simulink model "ValvingPTO"  (R2024b)
settings: Solver=VariableStepAuto  StartTime=0.0  StopTime=10.0  RelTol=1e-3
values from neighbouring files (symbols this model uses):
  params = struct    [BranchAndBound.m]    (also in Optimization.m; Parameters.m = struct(); RectangularOptimization.m; RoundingPI.m)
settings Model: Creator=jackson  LastModifiedBy=jackson

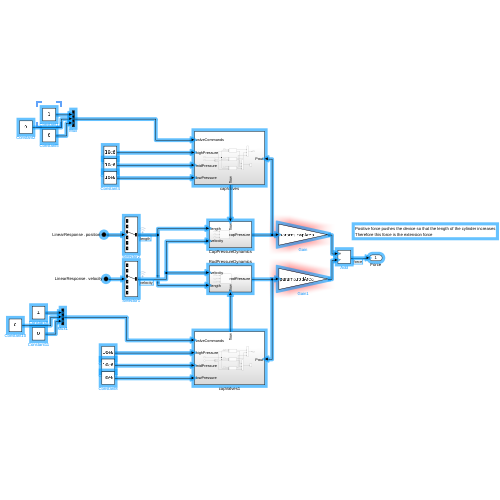
[thumbnail: Simulink's stored preview of the top-level diagram]
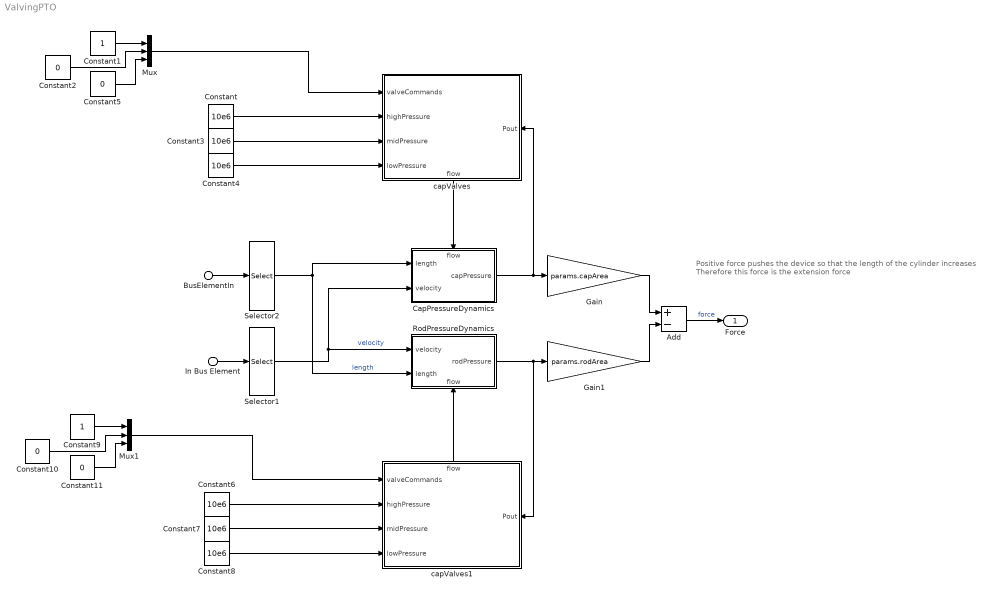
== system ValvingPTO ==
  note: Positive force pushes the device so that the length of the cylinder increases
      | Therefore this force is the extension force
  In Bus Element : Inport  PortName=LinearResponse  Element=velocity
  BusElementIn : Inport  PortName=LinearResponse  Element=position
  Add : Sum  Inputs=+-
  CapPressureDynamics : Subsystem
      settings: PortSchema="{\"entries\":[{\"content\":{\"sides\":[{\"content\":{\"connectorIds\":[\"In1\",\"In2\"]},\"type\":\"ConnectorPlacement.EquallySpacedRectSide\",\"uuid\":\"0a444e4d-7364-44e5-8b72-8c210fabafa0\"},{\"content\":{\"connectorIds\":[\"Out1\"],\"side\":\"RIGHT\"},\"type\":\"ConnectorPlacement.EquallySpacedRectSide\",\"uuid\":\"a3669697-8e2e-4fce-83e7-11feb3c41a11\"},{\"content\":{\"connectorIds\":[\"In3\"],\"side\":\"TOP\"},\"type\":\"ConnectorPlacement.EquallySpacedRectSide\",\"uuid\":\"edbd7469-179d-4b36-ab80-dceaa86ef763\"},{\"content\":{\"side\":\"BOTTOM\"},\"type\":\"ConnectorPlacement.EquallySpacedRectSide\",\"uuid\":\"36ba3990-6628-4e3d-ab1a-10917dd4fa0b\"}]},\"type\":\"ConnectorPlacement.EquallySpacedConnector\",\"uuid\":\"68480e3c-12c2-4c1a-9580-60c15ea9a162\"}],\"packageUris\":[\"http://schema.mathworks.com/mf0/Connector/R2020b\"],\"version\":\"1.0\"}"
  Constant{,3..4,6..8} (6 alike) : Constant  Value=10e6
  Constant1 : Constant
  Constant{2,5,10..11} (4 alike) : Constant  Value=0
  Constant9 : Constant
  Gain : Gain  Gain=params.capArea
  Gain1 : Gain  Gain=params.rodArea
  Mux : Mux  Inputs=3
  Mux1 : Mux  Inputs=3
  RodPressureDynamics : Subsystem
      settings: PortSchema="{\"entries\":[{\"content\":{\"sides\":[{\"content\":{\"connectorIds\":[\"In1\",\"In2\"]},\"type\":\"ConnectorPlacement.EquallySpacedRectSide\",\"uuid\":\"0a444e4d-7364-44e5-8b72-8c210fabafa0\"},{\"content\":{\"connectorIds\":[\"Out1\"],\"side\":\"RIGHT\"},\"type\":\"ConnectorPlacement.EquallySpacedRectSide\",\"uuid\":\"a3669697-8e2e-4fce-83e7-11feb3c41a11\"},{\"content\":{\"side\":\"TOP\"},\"type\":\"ConnectorPlacement.EquallySpacedRectSide\",\"uuid\":\"edbd7469-179d-4b36-ab80-dceaa86ef763\"},{\"content\":{\"connectorIds\":[\"In3\"],\"side\":\"BOTTOM\"},\"type\":\"ConnectorPlacement.EquallySpacedRectSide\",\"uuid\":\"0057cc85-602f-4ff7-8e06-c43254199496\"}]},\"type\":\"ConnectorPlacement.EquallySpacedConnector\",\"uuid\":\"68480e3c-12c2-4c1a-9580-60c15ea9a162\"}],\"packageUris\":[\"http://schema.mathworks.com/mf0/Connector/R2020b\"],\"version\":\"1.0\"}"
  Selector1 : Selector  InputPortWidth=6  IndexOptions=Index vector (dialog)  Indices=3  OutputSizes=1
  Selector2 : Selector  InputPortWidth=6  IndexOptions=Index vector (dialog)  Indices=3  OutputSizes=1
  capValves : Subsystem
      settings: PortSchema="{\"entries\":[{\"content\":{\"sides\":[{\"content\":{\"connectorIds\":[\"In1\",\"In2\",\"In3\",\"In4\"]},\"type\":\"ConnectorPlacement.EquallySpacedRectSide\",\"uuid\":\"d2e8cfa0-a0ae-49da-8fda-082dfd3b2d9f\"},{\"content\":{\"connectorIds\":[\"In5\"],\"side\":\"RIGHT\"},\"type\":\"ConnectorPlacement.EquallySpacedRectSide\",\"uuid\":\"7b83af61-76d6-4e35-9365-fafdba130762\"},{\"content\":{\"side\":\"TOP\"},\"type\":\"ConnectorPlacement.EquallySpacedRectSide\",\"uuid\":\"6880d985-ed9d-415d-a1a9-fc8aaf1ae9e0\"},{\"content\":{\"connectorIds\":[\"Out1\"],\"side\":\"BOTTOM\"},\"type\":\"ConnectorPlacement.EquallySpacedRectSide\",\"uuid\":\"f70b92c7-c6bf-4dbf-a331-364ba55ce8fb\"}]},\"type\":\"ConnectorPlacement.EquallySpacedConnector\",\"uuid\":\"7ffcaf2b-fb7f-4cb0-b739-43ebea45fc90\"}],\"packageUris\":[\"http://schema.mathworks.com/mf0/Connector/R2020b\"],\"version\":\"1.0\"}"
  capValves1 : Subsystem
      settings: PortSchema="{\"entries\":[{\"content\":{\"sides\":[{\"content\":{\"connectorIds\":[\"In1\",\"In2\",\"In3\",\"In4\"]},\"type\":\"ConnectorPlacement.EquallySpacedRectSide\",\"uuid\":\"d2e8cfa0-a0ae-49da-8fda-082dfd3b2d9f\"},{\"content\":{\"connectorIds\":[\"In5\"],\"side\":\"RIGHT\"},\"type\":\"ConnectorPlacement.EquallySpacedRectSide\",\"uuid\":\"7b83af61-76d6-4e35-9365-fafdba130762\"},{\"content\":{\"connectorIds\":[\"Out1\"],\"side\":\"TOP\"},\"type\":\"ConnectorPlacement.EquallySpacedRectSide\",\"uuid\":\"6880d985-ed9d-415d-a1a9-fc8aaf1ae9e0\"},{\"content\":{\"side\":\"BOTTOM\"},\"type\":\"ConnectorPlacement.EquallySpacedRectSide\",\"uuid\":\"f70b92c7-c6bf-4dbf-a331-364ba55ce8fb\"}]},\"type\":\"ConnectorPlacement.EquallySpacedConnector\",\"uuid\":\"7ffcaf2b-fb7f-4cb0-b739-43ebea45fc90\"}],\"packageUris\":[\"http://schema.mathworks.com/mf0/Connector/R2020b\"],\"version\":\"1.0\"}"
  Force : Outport
  wires:
  Add/1 -> Force/1  "force"
  BusElementIn/1 -> Selector2/1
  Selector1/1 -> RodPressureDynamics/1(velocity), CapPressureDynamics/2(velocity)  "velocity"
  Selector2/1 -> RodPressureDynamics/2(length), CapPressureDynamics/1(length)  "length"
  In Bus Element/1 -> Selector1/1
  Gain/1 -> Add/1
  Gain1/1 -> Add/2
  RodPressureDynamics/1(rodPressure) -> capValves1/5(Pout), Gain1/1
  CapPressureDynamics/1(capPressure) -> capValves/5(Pout), Gain/1
  Constant/1 -> capValves/2(highPressure)
  capValves/1(flow) -> CapPressureDynamics/3(flow)
  Constant1/1 -> Mux/1
  Constant2/1 -> Mux/2
  Mux/1 -> capValves/1(valveCommands)
  Constant3/1 -> capValves/3(midPressure)
  Constant4/1 -> capValves/4(lowPressure)
  Constant5/1 -> Mux/3
  capValves1/1(flow) -> RodPressureDynamics/3(flow)
  Constant8/1 -> capValves1/4(lowPressure)
  Constant6/1 -> capValves1/2(highPressure)
  Constant7/1 -> capValves1/3(midPressure)
  Constant9/1 -> Mux1/1
  Constant11/1 -> Mux1/3
  Mux1/1 -> capValves1/1(valveCommands)
  Constant10/1 -> Mux1/2

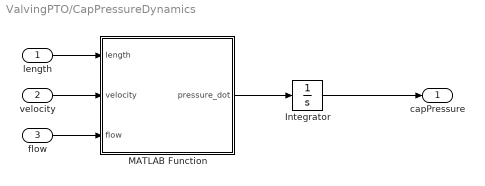
== system ValvingPTO/CapPressureDynamics ==
  length : Inport
  velocity : Inport  Port=2
  flow : Inport  Port=3
  Integrator : Integrator
  MATLAB Function : MATLAB Function  TreatAsAtomicUnit=on
  capPressure : Outport
  wires:
  MATLAB Function/1(pressure_dot) -> Integrator/1
  Integrator/1 -> capPressure/1
  flow/1 -> MATLAB Function/3(flow)
  velocity/1 -> MATLAB Function/2(velocity)
  length/1 -> MATLAB Function/1(length)

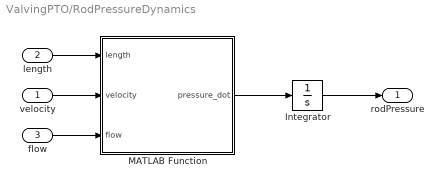
== system ValvingPTO/RodPressureDynamics ==
  velocity : Inport
  length : Inport  Port=2
  flow : Inport  Port=3
  Integrator : Integrator
  MATLAB Function : MATLAB Function  TreatAsAtomicUnit=on
  rodPressure : Outport
  wires:
  length/1 -> MATLAB Function/1(length)
  velocity/1 -> MATLAB Function/2(velocity)
  flow/1 -> MATLAB Function/3(flow)
  Integrator/1 -> rodPressure/1
  MATLAB Function/1(pressure_dot) -> Integrator/1

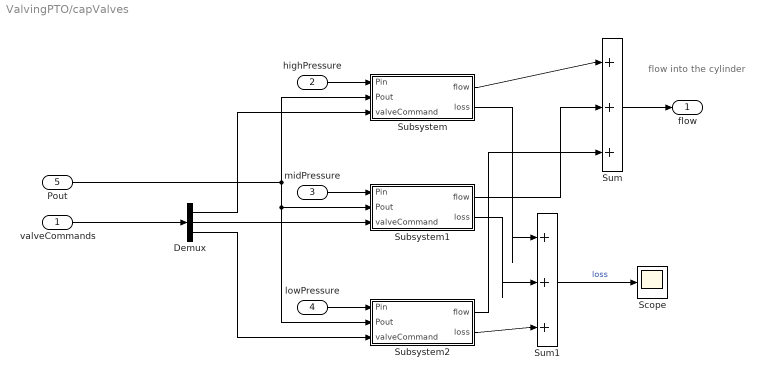
== system ValvingPTO/capValves ==
  note: flow into the cylinder
  valveCommands : Inport
  highPressure : Inport  Port=2
  midPressure : Inport  Port=3
  lowPressure : Inport  Port=4
  Pout : Inport  Port=5
  Demux : Demux  Outputs=3
  Scope : Scope
  Subsystem : Subsystem
  Subsystem1 : Subsystem
  Subsystem2 : Subsystem
  Sum : Sum  Inputs=|+++
  Sum1 : Sum  Inputs=|+++
  flow : Outport
  wires:
  Pout/1 -> Subsystem/2(Pout), Subsystem2/2(Pout), Subsystem1/2(Pout)
  highPressure/1 -> Subsystem/1(Pin)
  valveCommands/1 -> Demux/1
  Demux/1 -> Subsystem/3(valveCommand)
  midPressure/1 -> Subsystem1/1(Pin)
  lowPressure/1 -> Subsystem2/1(Pin)
  Demux/2 -> Subsystem1/3(valveCommand)
  Demux/3 -> Subsystem2/3(valveCommand)
  Subsystem/1(flow) -> Sum/1
  Subsystem1/1(flow) -> Sum/2
  Subsystem2/1(flow) -> Sum/3
  Sum/1 -> flow/1
  Subsystem/2(loss) -> Sum1/1
  Subsystem1/2(loss) -> Sum1/2
  Subsystem2/2(loss) -> Sum1/3
  Sum1/1 -> Scope/1  "loss"

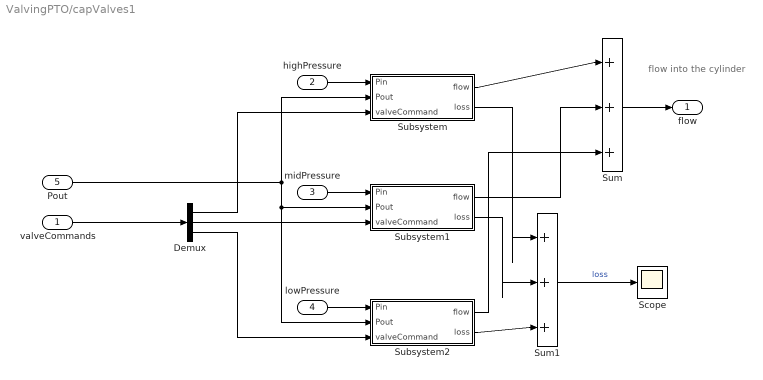
== system ValvingPTO/capValves1 ==
  note: flow into the cylinder
  valveCommands : Inport
  highPressure : Inport  Port=2
  midPressure : Inport  Port=3
  lowPressure : Inport  Port=4
  Pout : Inport  Port=5
  Demux : Demux  Outputs=3
  Scope : Scope
  Subsystem : Subsystem
  Subsystem1 : Subsystem
  Subsystem2 : Subsystem
  Sum : Sum  Inputs=|+++
  Sum1 : Sum  Inputs=|+++
  flow : Outport
  wires:
  Pout/1 -> Subsystem/2(Pout), Subsystem2/2(Pout), Subsystem1/2(Pout)
  highPressure/1 -> Subsystem/1(Pin)
  valveCommands/1 -> Demux/1
  Demux/1 -> Subsystem/3(valveCommand)
  midPressure/1 -> Subsystem1/1(Pin)
  lowPressure/1 -> Subsystem2/1(Pin)
  Demux/2 -> Subsystem1/3(valveCommand)
  Demux/3 -> Subsystem2/3(valveCommand)
  Subsystem/1(flow) -> Sum/1
  Subsystem1/1(flow) -> Sum/2
  Subsystem2/1(flow) -> Sum/3
  Sum/1 -> flow/1
  Subsystem/2(loss) -> Sum1/1
  Subsystem1/2(loss) -> Sum1/2
  Subsystem2/2(loss) -> Sum1/3
  Sum1/1 -> Scope/1  "loss"

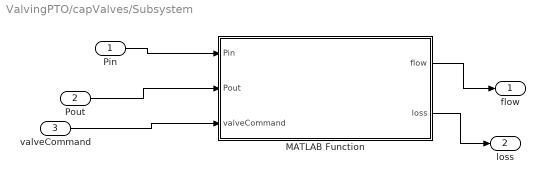
== system ValvingPTO/capValves/Subsystem ==
  Pin : Inport
  Pout : Inport  Port=2
  valveCommand : Inport  Port=3
  MATLAB Function : MATLAB Function  TreatAsAtomicUnit=on
  flow : Outport
  loss : Outport  Port=2
  wires:
  MATLAB Function/1(flow) -> flow/1
  valveCommand/1 -> MATLAB Function/3(valveCommand)
  Pout/1 -> MATLAB Function/2(Pout)
  Pin/1 -> MATLAB Function/1(Pin)
  MATLAB Function/2(loss) -> loss/1

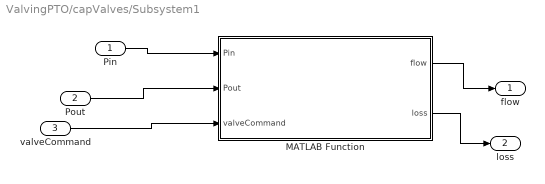
== system ValvingPTO/capValves/Subsystem1 ==
  Pin : Inport
  Pout : Inport  Port=2
  valveCommand : Inport  Port=3
  MATLAB Function : MATLAB Function  TreatAsAtomicUnit=on
  flow : Outport
  loss : Outport  Port=2
  wires:
  MATLAB Function/1(flow) -> flow/1
  valveCommand/1 -> MATLAB Function/3(valveCommand)
  Pout/1 -> MATLAB Function/2(Pout)
  Pin/1 -> MATLAB Function/1(Pin)
  MATLAB Function/2(loss) -> loss/1

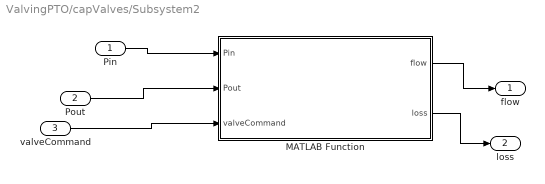
== system ValvingPTO/capValves/Subsystem2 ==
  Pin : Inport
  Pout : Inport  Port=2
  valveCommand : Inport  Port=3
  MATLAB Function : MATLAB Function  TreatAsAtomicUnit=on
  flow : Outport
  loss : Outport  Port=2
  wires:
  MATLAB Function/1(flow) -> flow/1
  valveCommand/1 -> MATLAB Function/3(valveCommand)
  Pout/1 -> MATLAB Function/2(Pout)
  Pin/1 -> MATLAB Function/1(Pin)
  MATLAB Function/2(loss) -> loss/1

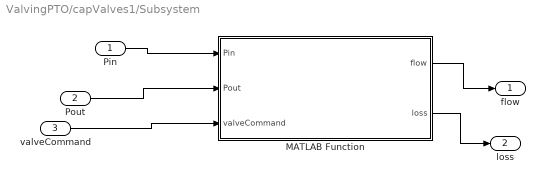
== system ValvingPTO/capValves1/Subsystem ==
  Pin : Inport
  Pout : Inport  Port=2
  valveCommand : Inport  Port=3
  MATLAB Function : MATLAB Function  TreatAsAtomicUnit=on
  flow : Outport
  loss : Outport  Port=2
  wires:
  MATLAB Function/1(flow) -> flow/1
  valveCommand/1 -> MATLAB Function/3(valveCommand)
  Pout/1 -> MATLAB Function/2(Pout)
  Pin/1 -> MATLAB Function/1(Pin)
  MATLAB Function/2(loss) -> loss/1

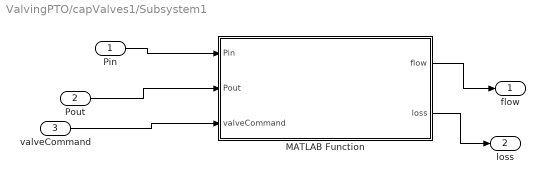
== system ValvingPTO/capValves1/Subsystem1 ==
  Pin : Inport
  Pout : Inport  Port=2
  valveCommand : Inport  Port=3
  MATLAB Function : MATLAB Function  TreatAsAtomicUnit=on
  flow : Outport
  loss : Outport  Port=2
  wires:
  MATLAB Function/1(flow) -> flow/1
  valveCommand/1 -> MATLAB Function/3(valveCommand)
  Pout/1 -> MATLAB Function/2(Pout)
  Pin/1 -> MATLAB Function/1(Pin)
  MATLAB Function/2(loss) -> loss/1

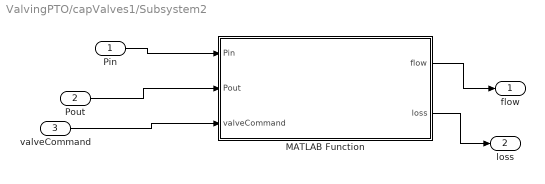
== system ValvingPTO/capValves1/Subsystem2 ==
  Pin : Inport
  Pout : Inport  Port=2
  valveCommand : Inport  Port=3
  MATLAB Function : MATLAB Function  TreatAsAtomicUnit=on
  flow : Outport
  loss : Outport  Port=2
  wires:
  MATLAB Function/1(flow) -> flow/1
  valveCommand/1 -> MATLAB Function/3(valveCommand)
  Pout/1 -> MATLAB Function/2(Pout)
  Pin/1 -> MATLAB Function/1(Pin)
  MATLAB Function/2(loss) -> loss/1

== matlab function ValvingPTO/RodPressureDynamics/MATLAB Function ==
  data: length input; velocity input; pressure_dot output; flow input; params parameter
function pressure_dot = RodPressure(length,velocity,flow,params)
% This code calculates the pressure dynamics on the rod side of the cylinder
% flow is flow into the rod side from the valves
% rod side is connected to the flap, positive velocity is extension

% get position from length. Position is measured from fully retracted.
% Positive is in extention
position = length - params.cylinderStroke; 

volume = params.capArea*( params.cylinderStroke - position);
pressure_dot = params.beta/volume * (flow - velocity*params.rodArea);

== matlab function ValvingPTO/CapPressureDynamics/MATLAB Function ==
  data: length input; velocity input; pressure_dot output; flow input; params parameter
function pressure_dot = CapPressure(length,velocity,flow,params)
% This code calculates the pressure dynamics on the cap side of the cylinder
% flow is flow into the cap side from the valves
% rod side is connected to the flap, positive velocity is extension

% get position from length. Position is measured from fully retracted.
% Positive is in extention
position = length - params.cylinderStroke; 

volume = params.capArea*position;
pressure_dot = params.beta/volume * (flow + velocity*params.capArea);

== matlab function ValvingPTO/capValves/Subsystem/MATLAB Function ==
  data: Pin input; flow output; Pout input; valveCommand input; params parameter; loss output
function [flow,loss] = fcn(Pin,Pout,valveCommand,params)

flow = valveCommand*params.valveConstant*sqrt(abs(Pout-Pin))*sign(Pout-Pin);
loss = (Pout-Pin)*flow;

== matlab function ValvingPTO/capValves/Subsystem1/MATLAB Function ==
  data: Pin input; flow output; Pout input; valveCommand input; params parameter; loss output
function [flow,loss] = fcn(Pin,Pout,valveCommand,params)

flow = valveCommand*params.valveConstant*sqrt(abs(Pout-Pin))*sign(Pout-Pin);
loss = (Pout-Pin)*flow;

== matlab function ValvingPTO/capValves/Subsystem2/MATLAB Function ==
  data: Pin input; flow output; Pout input; valveCommand input; params parameter; loss output
function [flow,loss] = fcn(Pin,Pout,valveCommand,params)

flow = valveCommand*params.valveConstant*sqrt(abs(Pout-Pin))*sign(Pout-Pin);
loss = (Pout-Pin)*flow;

== matlab function ValvingPTO/capValves1/Subsystem/MATLAB Function ==
  data: Pin input; flow output; Pout input; valveCommand input; params parameter; loss output
function [flow,loss] = fcn(Pin,Pout,valveCommand,params)

flow = valveCommand*params.valveConstant*sqrt(abs(Pout-Pin))*sign(Pout-Pin);
loss = (Pout-Pin)*flow;

== matlab function ValvingPTO/capValves1/Subsystem1/MATLAB Function ==
  data: Pin input; flow output; Pout input; valveCommand input; params parameter; loss output
function [flow,loss] = fcn(Pin,Pout,valveCommand,params)

flow = valveCommand*params.valveConstant*sqrt(abs(Pout-Pin))*sign(Pout-Pin);
loss = (Pout-Pin)*flow;

== matlab function ValvingPTO/capValves1/Subsystem2/MATLAB Function ==
  data: Pin input; flow output; Pout input; valveCommand input; params parameter; loss output
function [flow,loss] = fcn(Pin,Pout,valveCommand,params)

flow = valveCommand*params.valveConstant*sqrt(abs(Pout-Pin))*sign(Pout-Pin);
loss = (Pout-Pin)*flow;
